simulink model "PerturbatiePeIntrare"  (R2023b)
settings: Solver=VariableStepAuto  StartTime=0.0  StopTime=1000  RelTol=1e-3
values from neighbouring files (symbols this model uses):
  k = 0.036    [date_personalizate.m]    (also in grafice.m = 0.035)
  k1 = 0.624    [date_personalizate.m]    (also in grafice.m)
  k2 = -0.015    [date_personalizate.m]    (also in grafice.m)
  k3 = -0.0006    [date_personalizate.m]    (also in grafice.m)
  keta = 8e-5    (= 8e-05)    [date_personalizate.m]
libraries: slpidlib x1
settings Model: Creator=40787  LastModifiedBy=40787

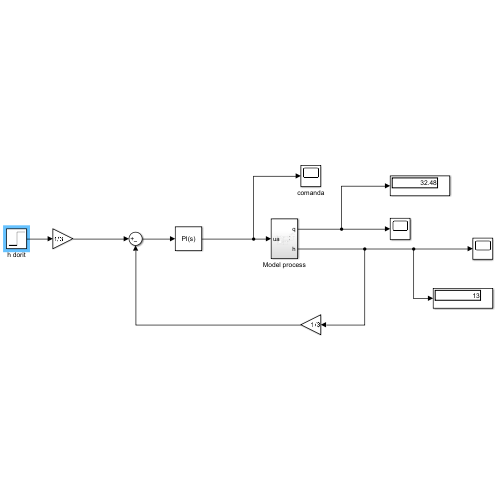
[thumbnail: Simulink's stored preview of the top-level diagram]
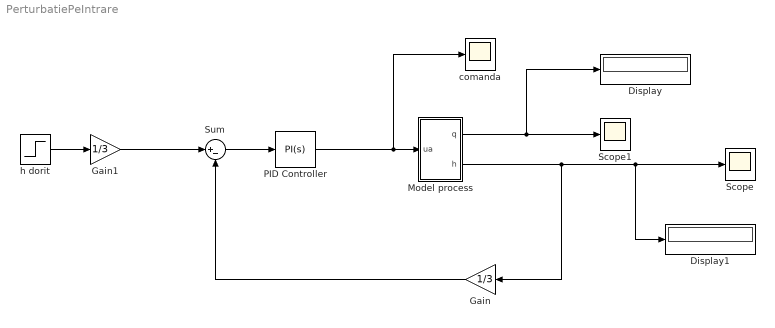
== system PerturbatiePeIntrare ==
  Display : Display
  Display1 : Display
  Gain : Gain  Gain=1/3
  Gain1 : Gain  Gain=1/3
  Model process : Subsystem
  PID Controller : slpidlib/PID Controller  Controller=PI  Form=Parallel  TimeDomain=Continuous-time  UseExternalTs=off  SampleTime=-1  IntegratorMethod=Forward Euler  FilterMethod=Forward Euler  ControllerParametersSource=internal  P=2.395  I=2.395/159  UseKiTs=off  D=0  N=100  UseFilter=on  TunerSelectOption=Frequency Response Based  InitialConditionSource=internal  InitialConditionForIntegrator=5  InitialConditionForFilter=0  DifferentiatorICPrevScaledInput=0  ExternalReset=none  TrackingMode=off  Kt=1  LimitOutput=off  SatLimitsSource=internal  UpperSaturationLimit=inf  LowerSaturationLimit=-inf  LinearizeAsGain=on  AntiWindupMode=none  Kb=1  LimitIntegrator=off  UpperIntegratorSaturationLimit=inf  LowerIntegratorSaturationLimit=-inf  POutMin=[]  POutMax=[]  IOutMin=[]  IOutMax=[]  DOutMin=[]  DOutMax=[]  NOutMin=[]  NOutMax=[]  SumOutMin=[]  SumOutMax=[]  SaturationOutMin=[]  SaturationOutMax=[]  PParamMin=[]  PParamMax=[]  IParamMin=[]  IParamMax=[]  DParamMin=[]  DParamMax=[]  NParamMin=[]  NParamMax=[]  KbParamMin=[]  KbParamMax=[]  KtParamMin=[]  KtParamMax=[]  KbOutMin=[]  KbOutMax=[]  KtOutMin=[]  KtOutMax=[]  IntegratorOutMin=[]  IntegratorOutMax=[]  FilterOutMin=[]  FilterOutMax=[]  SumI1OutMin=[]  SumI1OutMax=[]  SumI2OutMin=[]  SumI2OutMax=[]  SumI3OutMin=[]  SumI3OutMax=[]  SumI4OutMin=[]  SumI4OutMax=[]  SumDOutMin=[]  SumDOutMax=[]  DifferentiatorOutMin=[]  DifferentiatorOutMax=[]  FilterDiffOutCoefMin=[]  FilterDiffOutCoefMax=[]  ReciprocalOutMin=[]  ReciprocalOutMax=[]  SumDenOutMin=[]  SumDenOutMax=[]  SumNumOutMin=[]  SumNumOutMax=[]  DivideOutMin=[]  DivideOutMax=[]  UdiffTsProdOutMin=[]  UdiffTsProdOutMax=[]  NTsProdOutMin=[]  NTsProdOutMax=[]  UintegralTsProdOutMin=[]  UintegralTsProdOutMax=[]  UngainTsProdOutMin=[]  UngainTsProdOutMax=[]  ClampingZeroOutDataTypeStr=Inherit: Inherit via back propagation  ClampingZeroOutMin=[]  ClampingZeroOutMax=[]  FilterDenConstantOutDataTypeStr=Inherit: Inherit via back propagation  FilterDenConstantOutMin=[]  FilterDenConstantOutMax=[]  PCopyOutDataTypeStr=Inherit: Inherit via back propagation  PCopyOutMin=[]  PCopyOutMax=[]  NCopyOutDataTypeStr=Inherit: Inherit via back propagation  NCopyOutMin=[]  NCopyOutMax=[]  IntegratorContinuousStateAttributes=''  IntegratorStateMustResolveToSignalObject=off  IntegratorRTWStateStorageClass=Auto  FilterContinuousStateAttributes=''  FilterStateMustResolveToSignalObject=off  FilterRTWStateStorageClass=Auto  ParallelPVariant=InternalParameters  IdealPVariant=Disabled  IVariant=InternalParameters  DVariant=Disabled  IntegratorVariant=Continuous  SatVariant=Disabled  AWVariant=Passthrough  PCopyVariant=Disabled  TRVariant=Disabled  FdbkBlocksVariant=Forward  IdealPFdbkVariant=Disabled  SatFdbkVariant=Disabled  DerivativeFilterVariant=Disabled  NVariant=Disabled  NCopyVariant=Disabled_SignalSpec  FilterICVariant=Disabled  IntegratorICVariant=InternalICs  ExternalResetVariant=Disabled  TRSumVariant=Passthrough  SumFdbkVariant=Disabled  SumVariant=Sum_PI  TsampFilterVariant=InternalTs  TsampNgainVariant=Passthrough  TsampIntegralVariant=Disabled_SignalSpec  ExternalSaturationOutDataTypeStr=Inherit: Same as second input
  Scope : Scope
  Scope1 : Scope
  Sum : Sum  Inputs=|+-
  comanda : Scope
  h dorit : Step  Time=0  After=13  SampleTime=0
  wires:
  Gain/1 -> Sum/2
  PID Controller/1 -> comanda/1, Model process/1(ua)
  h dorit/1 -> Gain1/1
  Gain1/1 -> Sum/1
  Sum/1 -> PID Controller/1
  Model process/2(h) -> Display1/1, Scope/1, Gain/1
  Model process/1(q) -> Display/1, Scope1/1

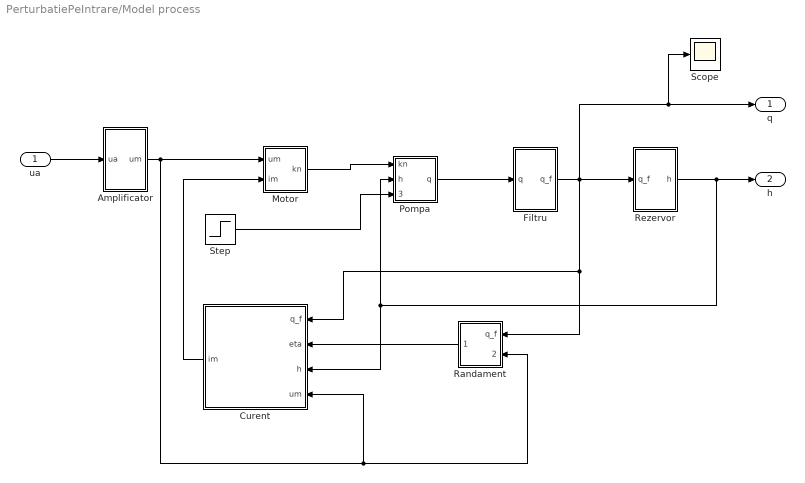
== system PerturbatiePeIntrare/Model process ==
  ua : Inport
  "Amplificator " : Subsystem
  Curent : Subsystem
  Filtru : Subsystem
  Motor : Subsystem
  Pompa : Subsystem
  Randament : Subsystem
  Rezervor : Subsystem
  Scope : Scope
  Step : Step  Time=300  After=0.006  SampleTime=0
  q : Outport
  h : Outport  Port=2
  wires:
  ua/1 -> "Amplificator "/1(ua)
  Motor/1(kn) -> Pompa/1(kn)
  "Amplificator "/1(um) -> Curent/4(um), Randament/2(um), Motor/1(um)
  Rezervor/1(h) -> h/1, Curent/3(h), Pompa/2(h)
  Curent/1(im) -> Motor/2(im)
  Filtru/1(q_f) -> Rezervor/1(q_f), Scope/1, q/1, Curent/1(q_f), Randament/1(q_f)
  Randament/1(eta) -> Curent/2(eta)
  Pompa/1(q) -> Filtru/1(q)
  Step/1 -> Pompa/3(perturbatia k)

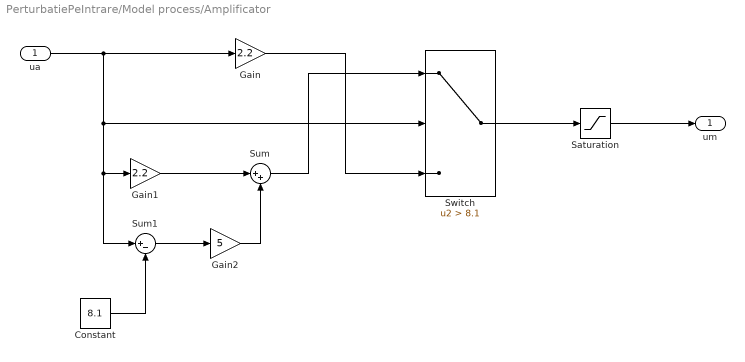
== system PerturbatiePeIntrare/Model process/Amplificator  ==
  ua : Inport
  Constant : Constant  Value=8.1
  Gain : Gain  Gain=2.2
  Gain1 : Gain  Gain=2.2
  Gain2 : Gain  Gain=5
  Saturation : Saturate  UpperLimit=22  LowerLimit=0
  Sum : Sum  Inputs=|++
  Sum1 : Sum  Inputs=|+-
  Switch : Switch  Criteria=u2 > Threshold  Threshold=8.1  SaturateOnIntegerOverflow=off  InputSameDT=off
  um : Outport
  wires:
  Gain2/1 -> Sum/2
  Gain1/1 -> Sum/1
  Sum1/1 -> Gain2/1
  Sum/1 -> Switch/1
  ua/1 -> Gain/1, Gain1/1, Sum1/1, Switch/2
  Constant/1 -> Sum1/2
  Gain/1 -> Switch/3
  Switch/1 -> Saturation/1
  Saturation/1 -> um/1

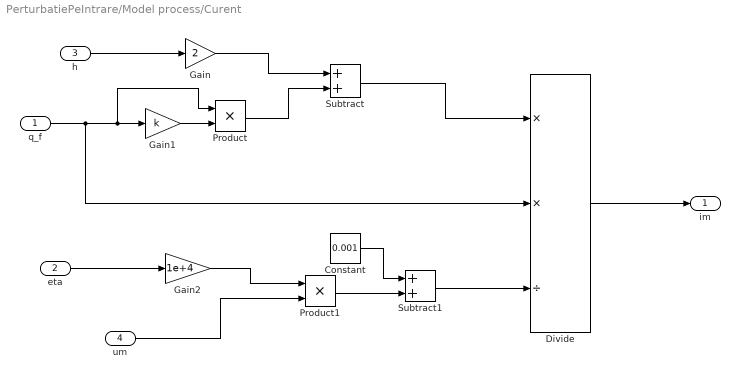
== system PerturbatiePeIntrare/Model process/Curent ==
  q_f : Inport
  eta : Inport  Port=2
  h : Inport  Port=3
  um : Inport  Port=4
  Constant : Constant  Value=0.001
  Divide : Product  Inputs=**/
  Gain : Gain  Gain=2
  Gain1 : Gain  Gain=k
  Gain2 : Gain  Gain=1e+4
  Product : Product
  Product1 : Product
  Subtract : Sum
  Subtract1 : Sum
  im : Outport
  wires:
  um/1 -> Product1/2
  h/1 -> Gain/1
  Product1/1 -> Subtract1/2
  eta/1 -> Gain2/1
  Gain/1 -> Subtract/1
  Constant/1 -> Subtract1/1
  Subtract/1 -> Divide/1
  Gain2/1 -> Product1/1
  Product/1 -> Subtract/2
  Subtract1/1 -> Divide/3
  q_f/1 -> Product/1, Gain1/1, Divide/2
  Divide/1 -> im/1
  Gain1/1 -> Product/2

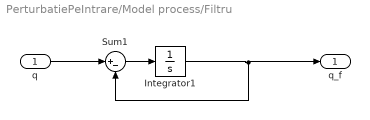
== system PerturbatiePeIntrare/Model process/Filtru ==
  q : Inport
  Integrator1 : Integrator  InitialCondition=29.18
  Sum1 : Sum  Inputs=|+-
  q_f : Outport
  wires:
  Sum1/1 -> Integrator1/1
  Integrator1/1 -> q_f/1, Sum1/2
  q/1 -> Sum1/1

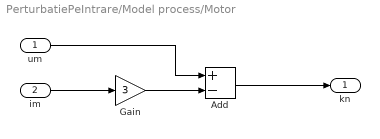
== system PerturbatiePeIntrare/Model process/Motor ==
  um : Inport
  im : Inport  Port=2
  Add : Sum  Inputs=+-
  Gain : Gain  Gain=3
  kn : Outport
  wires:
  Gain/1 -> Add/2
  im/1 -> Gain/1
  um/1 -> Add/1
  Add/1 -> kn/1

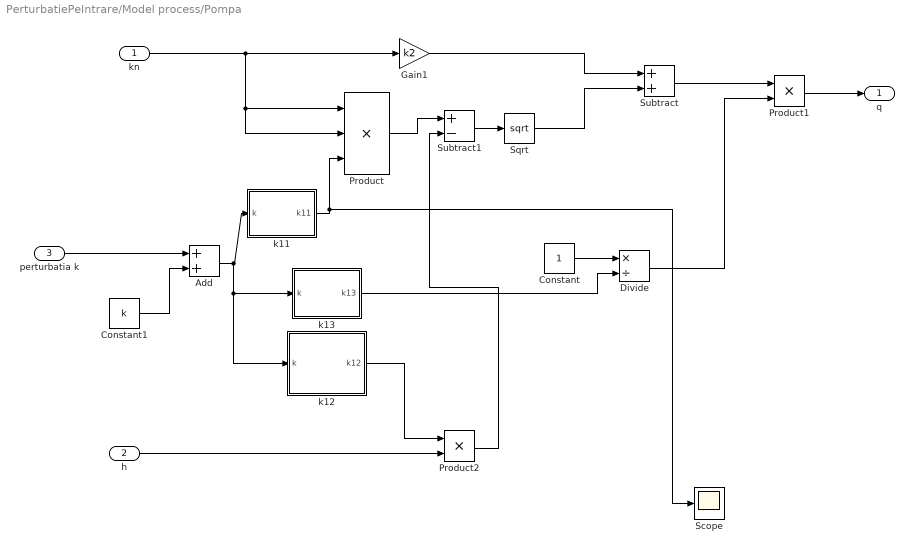
== system PerturbatiePeIntrare/Model process/Pompa ==
  kn : Inport
  h : Inport  Port=2
  perturbatia k : Inport  Port=3
  Add : Sum
  Constant : Constant
  Constant1 : Constant  Value=k
  Divide : Product  Inputs=*/
  Gain1 : Gain  Gain=k2
  Product : Product  Inputs=3
  Product1 : Product
  Product2 : Product
  Scope : Scope
  Sqrt : Sqrt
  Subtract : Sum
  Subtract1 : Sum  Inputs=+-
  k11 : Subsystem
  k12 : Subsystem
  k13 : Subsystem
  q : Outport
  wires:
  Sqrt/1 -> Subtract/2
  kn/1 -> Product/2, Product/1, Gain1/1
  Subtract1/1 -> Sqrt/1
  Gain1/1 -> Subtract/1
  Product1/1 -> q/1
  Subtract/1 -> Product1/1
  Product/1 -> Subtract1/1
  perturbatia k/1 -> Add/1
  h/1 -> Product2/2
  Add/1 -> k12/1(k), k13/1(k), k11/1(k)
  k11/1(k11) -> Product/3, Scope/1
  Product2/1 -> Subtract1/2
  Constant/1 -> Divide/1
  k13/1(k13) -> Divide/2
  Divide/1 -> Product1/2
  Constant1/1 -> Add/2
  k12/1(k12) -> Product2/1

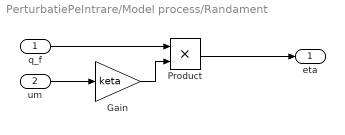
== system PerturbatiePeIntrare/Model process/Randament ==
  q_f : Inport
  um : Inport  Port=2
  Gain : Gain  Gain=keta
  Product : Product
  eta : Outport
  wires:
  Gain/1 -> Product/2
  um/1 -> Gain/1
  q_f/1 -> Product/1
  Product/1 -> eta/1

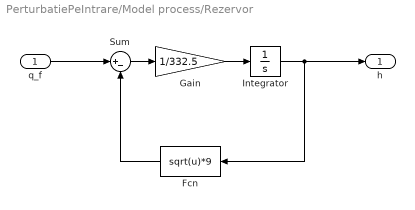
== system PerturbatiePeIntrare/Model process/Rezervor ==
  q_f : Inport
  Fcn : Fcn  Expr=sqrt(u)*9
  Gain : Gain  Gain=1/332.5
  Integrator : Integrator  InitialCondition=10.51
  Sum : Sum  Inputs=|+-
  h : Outport
  wires:
  Gain/1 -> Integrator/1
  q_f/1 -> Sum/1
  Integrator/1 -> h/1, Fcn/1
  Sum/1 -> Gain/1
  Fcn/1 -> Sum/2

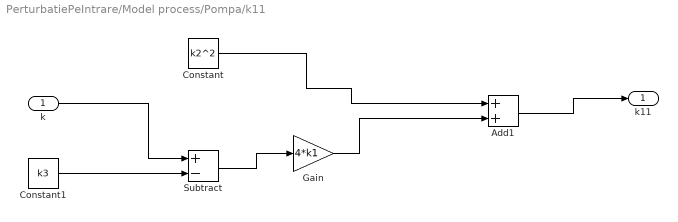
== system PerturbatiePeIntrare/Model process/Pompa/k11 ==
  k : Inport
  Add1 : Sum
  Constant : Constant  Value=k2^2
  Constant1 : Constant  Value=k3
  Gain : Gain  Gain=4*k1
  Subtract : Sum  Inputs=+-
  k11 : Outport
  wires:
  Add1/1 -> k11/1
  Gain/1 -> Add1/2
  Constant/1 -> Add1/1
  Constant1/1 -> Subtract/2
  k/1 -> Subtract/1
  Subtract/1 -> Gain/1

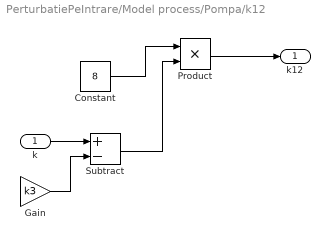
== system PerturbatiePeIntrare/Model process/Pompa/k12 ==
  k : Inport
  Constant : Constant  Value=8
  Gain : Gain  Gain=k3
  Product : Product
  Subtract : Sum  Inputs=+-
  k12 : Outport
  wires:
  Constant/1 -> Product/1
  k/1 -> Subtract/1
  Gain/1 -> Subtract/2
  Subtract/1 -> Product/2
  Product/1 -> k12/1

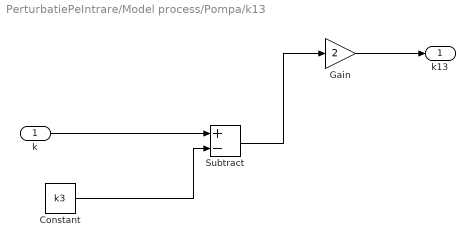
== system PerturbatiePeIntrare/Model process/Pompa/k13 ==
  k : Inport
  Constant : Constant  Value=k3
  Gain : Gain  Gain=2
  Subtract : Sum  Inputs=+-
  k13 : Outport
  wires:
  k/1 -> Subtract/1
  Gain/1 -> k13/1
  Constant/1 -> Subtract/2
  Subtract/1 -> Gain/1
